simulink model "scale_model_model_control"  (R2024b)
settings: Solver=VariableStepAuto  StartTime=0.0  StopTime=100  MaxStep=0.02  RelTol=1e-3
values from neighbouring files (symbols this model uses):
  A_adrcl = [zeros(N, 1)  eye(N, N) ... (first row only)    [init_scale_blade_suspended_control.m]
  A_ESO_d = [1-l1_ESO_d, delta_t-l1_ESO_d*delta_t, 1/2 * delta_t^2 - 1/2 * l1_ESO_d*delta_t^2 ... (first row only)    [init_scale_blade_suspended_control.m]
  A_MESO_d = A_o_d - l_MESO_d*C_o_d*A_o_d    [init_scale_blade_suspended_control.m]
  b0 = 1.025    [init_scale_blade_suspended_control.m]
  b_adrcl = [zeros(N-1, 1) ... (first row only)    [init_scale_blade_suspended_control.m]
  b_ESO_d = [1/2*b0*delta_t^2 - l1_ESO_d*b0*delta_t^2 ... (first row only)    [init_scale_blade_suspended_control.m]
  B_MESO_d = B_o_d - l_MESO_d*C_o_d*B_o_d    [init_scale_blade_suspended_control.m]
  c_t = [1, zeros(1, N)]    [init_scale_blade_suspended_control.m]
  delta_t = 0.01    [init_scale_blade_suspended_control.m]
  DLADRC_max_effort = 30    [init_scale_blade_suspended_control.m]
  DLQRMADRC_max_effort = 30    [init_scale_blade_suspended_control.m]
  eta_s_init_n = [p_s_init_n;Theta_s_init_n]    [init_scale_blade_suspended_control.m]
  g = 9.81    [init_scale_blade_suspended_control.m]
  inv_M_s = inv(M_s)    [init_scale_blade_suspended_control.m]
  k = ones(N,1)    [init_scale_blade_suspended_control.m]
  k1_c_d = (1 - z_cl)^2/delta_t^2    [init_scale_blade_suspended_control.m]
  k_c_T_dlqr = dlqr(A_m_dlqr,b_m_dlqr,Q,R)    [init_scale_blade_suspended_control.m]
  k_d_T_lqr = (e_m*c_T_d_m_lqr) \ b_m_lqr    [init_scale_blade_suspended_control.m]
  k_s_lqr = -inv(c_T_m_lqr*inv(A_m_lqr-b_m_lqr*k_c_T_lqr)*b_m_lqr)    [init_scale_blade_suspended_control.m]
  k_T_d = [k1_c_d, k2_c_d]    [init_scale_blade_suspended_control.m]
  k_w1_s = gamma * EA/lw1_s_init    (= 19634.9540849)    [init_scale_blade_suspended_control.m]
  k_w2_s = k_w1_s    (= 19634.9540849)    [init_scale_blade_suspended_control.m]
  L = 0.8    [init_scale_blade_suspended_control.m]
  l = ones(N+1, 1)    [init_scale_blade_suspended_control.m]
  l_ESO_d = [l1_ESO_d, l2_ESO_d, l3_ESO_d]'    [init_scale_blade_suspended_control.m]
  l_MESO_d = acker(A_o_d',C_o_d',[z_MESO,z_MESO,z_MESO])'    [init_scale_blade_suspended_control.m]
  lw1_s_init = tot_liftWire-0.14    (= 0.56)    [init_scale_blade_suspended_control.m]
  lw2_s = norm(p_h_s_init- posSling_s_n(:,1))-elong_lw2_s    [init_scale_blade_suspended_control.m]
  m_h_s = 0.01    [init_scale_blade_suspended_control.m]
  meanWSP = 1    [init_scale_blade_suspended_control.m]
  N = 2    [init_scale_blade_suspended_control.m]
  nu_s_init_b = zeros(6,1)    [init_scale_blade_suspended_control.m]
  p_h_dot_s_init = [0;0;0]    [init_scale_blade_suspended_control.m]
  p_h_s_init = posCraneTip_s + [0;0;lw1_s_init + elong_mainlw_s]    [init_scale_blade_suspended_control.m]
  posCOG_s = [0;0;0]    [init_scale_blade_suspended_control.m]
  posCraneTip_s = [0;0;-1.2]    [init_scale_blade_suspended_control.m]
  posSling_s_b = [posCOG_s + [slings_p1_new(1); -0.05; slings_p1_new(2)],                posCOG_s + [slings_p1_new(1); 0.05; slings_p1_new(2)],               posCOG_s + [slings_p2_new(1); -0.05; slings_p2_new(2)],               posCOG_s + [slings_p2_new(1); 0.05; slings_p2_new(2)]]    [init_scale_blade_suspended_control.m]
  posThruster_s_b = [posCOG_s + [0.03; 0.21; -0.05],                posCOG_s + [0.03; -0.21; -0.05],               posCOG_s + [0; 0.1825; -0.05],               posCOG_s + [0; -0.1825; -0.05]]    [init_scale_blade_suspended_control.m]
  totalMass_s = 0.391    [init_scale_blade_suspended_control.m]
  W = 0.05    [init_scale_blade_suspended_control.m]
undefined symbols (not defined in the file or in its folder): A_o_dlqr, b_o_dlqr, c_o_T_dlqr, k_o_lqr, linsys_v2, sigbuilder_block
libraries: MarIn_blade x104, simulink_extras x28, slpidlib x5, simulink x4
(part 1 of 3)
settings Model: Creator=Basti  LastModifiedBy=Henrik
settings DebuggingCC: UnconnectedInputMsg=warning  UnconnectedOutputMsg=warning  UnconnectedLineMsg=warning
settings ModelReferenceCC: EnableRefExpFcnMdlSchedulingChecks=on
settings RTWCC: GPUComputeCapability=3.5  DLArmComputeVersion=19.05

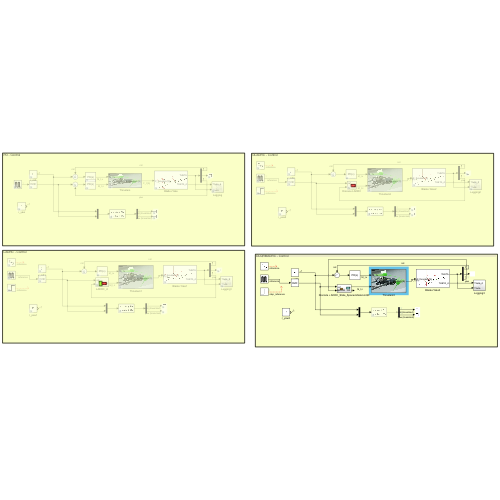
[thumbnail: Simulink's stored preview of the top-level diagram]
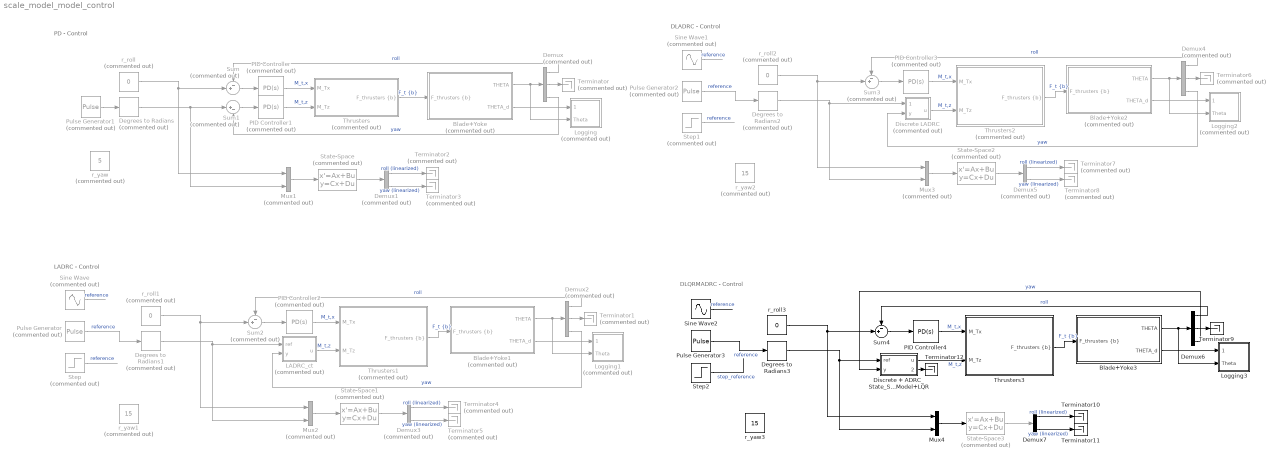
== system scale_model_model_control ==
  note: PD - Control
  note: LADRC - Control
  note: DLADRC - Control
  note: DLQRMADRC - Control
  Blade+Yoke : Subsystem  Commented=on
      mask Display: image('$imagefile'); % Use "Edit Image" on toolstrip to change.
  Blade+Yoke1 : Subsystem  Commented=on
      mask Display: image('$imagefile'); % Use "Edit Image" on toolstrip to change.
  Blade+Yoke2 : Subsystem  Commented=on
      mask Display: image('$imagefile'); % Use "Edit Image" on toolstrip to change.
  Blade+Yoke3 : Subsystem
      mask Display: image('$imagefile'); % Use "Edit Image" on toolstrip to change.
  Degrees to Radians : simulink_extras/Transformations/Degrees to Radians  Commented=on
  Degrees to Radians1 : simulink_extras/Transformations/Degrees to Radians  Commented=on
  Degrees to Radians2 : simulink_extras/Transformations/Degrees to Radians  Commented=on
  Degrees to Radians3 : simulink_extras/Transformations/Degrees to Radians
  Demux : Demux  Commented=on  Outputs=3
  Demux1 : Demux  Commented=on  Outputs=2
  Demux2 : Demux  Commented=on  Outputs=3
  Demux3 : Demux  Commented=on  Outputs=2
  Demux4 : Demux  Commented=on  Outputs=3
  Demux5 : Demux  Commented=on  Outputs=2
  Demux6 : Demux  Outputs=3
  Demux7 : Demux  Outputs=2
  Discrete + ADRC_State_Space+Model+LQR : Subsystem
  Discrete LADRC : Subsystem  Commented=on
  LADRC_ct : Subsystem  Commented=on
  Logging : Subsystem  Commented=on
  Logging1 : Subsystem  Commented=on
  Logging2 : Subsystem  Commented=on
  Logging3 : Subsystem
  Mux1 : Mux  Commented=on  Inputs=2
  Mux2 : Mux  Commented=on  Inputs=2
  Mux3 : Mux  Commented=on  Inputs=2
  Mux4 : Mux  Inputs=2
  PID Controller : slpidlib/PID Controller  Commented=on  Controller=PD  Form=Parallel  TimeDomain=Continuous-time  UseExternalTs=off  SampleTime=-1  IntegratorMethod=Forward Euler  FilterMethod=Forward Euler  ControllerParametersSource=internal  P=0.561459634219398  I=1  UseKiTs=off  D=0.260333020296235  UseExternalDerivativeSource=off  N=93.2588541333035  UseFilter=on  TunerSelectOption=Transfer Function Based (PID Tuner App)  InitialConditionSource=internal  InitialConditionForIntegrator=0  InitialConditionForFilter=0  DifferentiatorICPrevScaledInput=0  ExternalReset=none  TrackingMode=off  Kt=1  LimitOutput=off  SatLimitsSource=internal  UpperSaturationLimit=inf  LowerSaturationLimit=-inf  LinearizeAsGain=on  AntiWindupMode=none  Kb=1  LimitIntegrator=off  UpperIntegratorSaturationLimit=inf  LowerIntegratorSaturationLimit=-inf  POutMin=[]  POutMax=[]  IOutMin=[]  IOutMax=[]  DOutMin=[]  DOutMax=[]  NOutMin=[]  NOutMax=[]  SumOutMin=[]  SumOutMax=[]  SaturationOutMin=[]  SaturationOutMax=[]  PParamMin=[]  PParamMax=[]  IParamMin=[]  IParamMax=[]  DParamMin=[]  DParamMax=[]  NParamMin=[]  NParamMax=[]  KbParamMin=[]  KbParamMax=[]  KtParamMin=[]  KtParamMax=[]  KbOutMin=[]  KbOutMax=[]  KtOutMin=[]  KtOutMax=[]  IntegratorOutMin=[]  IntegratorOutMax=[]  FilterOutMin=[]  FilterOutMax=[]  SumI1OutMin=[]  SumI1OutMax=[]  SumI2OutMin=[]  SumI2OutMax=[]  SumI3OutMin=[]  SumI3OutMax=[]  SumI4OutMin=[]  SumI4OutMax=[]  SumDOutMin=[]  SumDOutMax=[]  DifferentiatorOutMin=[]  DifferentiatorOutMax=[]  FilterDiffOutCoefMin=[]  FilterDiffOutCoefMax=[]  ReciprocalOutMin=[]  ReciprocalOutMax=[]  SumDenOutMin=[]  SumDenOutMax=[]  SumNumOutMin=[]  SumNumOutMax=[]  DivideOutMin=[]  DivideOutMax=[]  UdiffTsProdOutMin=[]  UdiffTsProdOutMax=[]  NTsProdOutMin=[]  NTsProdOutMax=[]  UintegralTsProdOutMin=[]  UintegralTsProdOutMax=[]  UngainTsProdOutMin=[]  UngainTsProdOutMax=[]  ClampingZeroOutDataTypeStr=Inherit: Inherit via back propagation  ClampingZeroOutMin=[]  ClampingZeroOutMax=[]  FilterDenConstantOutDataTypeStr=Inherit: Inherit via back propagation  FilterDenConstantOutMin=[]  FilterDenConstantOutMax=[]  PCopyOutDataTypeStr=Inherit: Inherit via back propagation  PCopyOutMin=[]  PCopyOutMax=[]  NCopyOutDataTypeStr=Inherit: Inherit via back propagation  NCopyOutMin=[]  NCopyOutMax=[]  IntegratorContinuousStateAttributes=''  IntegratorStateMustResolveToSignalObject=off  IntegratorRTWStateStorageClass=Auto  FilterContinuousStateAttributes=''  FilterStateMustResolveToSignalObject=off  FilterRTWStateStorageClass=Auto  ParallelPVariant=InternalParameters  IdealPVariant=Disabled  IVariant=Disabled  DVariant=InternalParameters  IntegratorVariant=Disabled  SatVariant=Disabled  AWVariant=Disabled  PCopyVariant=Disabled  TRVariant=Disabled  FdbkBlocksVariant=Forward  IdealPFdbkVariant=Disabled  SatFdbkVariant=Disabled  DerivativeFilterVariant=ContFilter  NVariant=InternalParameters  NCopyVariant=Disabled  FilterICVariant=InternalICsFilter  IntegratorICVariant=Disabled  ExternalResetVariant=Disabled  TRSumVariant=Passthrough  SumFdbkVariant=Disabled  SumVariant=Sum_PD  TsampFilterVariant=InternalTs  TsampNgainVariant=Passthrough  TsampIntegralVariant=Disabled_SignalSpec  ExternalSaturationOutDataTypeStr=Inherit: Same as second input  DerivativeSourceVariant=ErrorSignal  PreIntVariant=InternalPreInt
  PID Controller1 : slpidlib/PID Controller  Commented=on  Controller=PD  Form=Parallel  TimeDomain=Continuous-time  UseExternalTs=off  SampleTime=-1  IntegratorMethod=Forward Euler  FilterMethod=Forward Euler  ControllerParametersSource=internal  P=12.7  I=1  UseKiTs=off  D=1.297*5  UseExternalDerivativeSource=off  N=6677.648  UseFilter=on  TunerSelectOption=Transfer Function Based (PID Tuner App)  InitialConditionSource=internal  InitialConditionForIntegrator=0  InitialConditionForFilter=0  DifferentiatorICPrevScaledInput=0  ExternalReset=none  TrackingMode=off  Kt=1  LimitOutput=off  SatLimitsSource=internal  UpperSaturationLimit=inf  LowerSaturationLimit=-inf  LinearizeAsGain=on  AntiWindupMode=none  Kb=1  LimitIntegrator=off  UpperIntegratorSaturationLimit=inf  LowerIntegratorSaturationLimit=-inf  POutMin=[]  POutMax=[]  IOutMin=[]  IOutMax=[]  DOutMin=[]  DOutMax=[]  NOutMin=[]  NOutMax=[]  SumOutMin=[]  SumOutMax=[]  SaturationOutMin=[]  SaturationOutMax=[]  PParamMin=[]  PParamMax=[]  IParamMin=[]  IParamMax=[]  DParamMin=[]  DParamMax=[]  NParamMin=[]  NParamMax=[]  KbParamMin=[]  KbParamMax=[]  KtParamMin=[]  KtParamMax=[]  KbOutMin=[]  KbOutMax=[]  KtOutMin=[]  KtOutMax=[]  IntegratorOutMin=[]  IntegratorOutMax=[]  FilterOutMin=[]  FilterOutMax=[]  SumI1OutMin=[]  SumI1OutMax=[]  SumI2OutMin=[]  SumI2OutMax=[]  SumI3OutMin=[]  SumI3OutMax=[]  SumI4OutMin=[]  SumI4OutMax=[]  SumDOutMin=[]  SumDOutMax=[]  DifferentiatorOutMin=[]  DifferentiatorOutMax=[]  FilterDiffOutCoefMin=[]  FilterDiffOutCoefMax=[]  ReciprocalOutMin=[]  ReciprocalOutMax=[]  SumDenOutMin=[]  SumDenOutMax=[]  SumNumOutMin=[]  SumNumOutMax=[]  DivideOutMin=[]  DivideOutMax=[]  UdiffTsProdOutMin=[]  UdiffTsProdOutMax=[]  NTsProdOutMin=[]  NTsProdOutMax=[]  UintegralTsProdOutMin=[]  UintegralTsProdOutMax=[]  UngainTsProdOutMin=[]  UngainTsProdOutMax=[]  ClampingZeroOutDataTypeStr=Inherit: Inherit via back propagation  ClampingZeroOutMin=[]  ClampingZeroOutMax=[]  FilterDenConstantOutDataTypeStr=Inherit: Inherit via back propagation  FilterDenConstantOutMin=[]  FilterDenConstantOutMax=[]  PCopyOutDataTypeStr=Inherit: Inherit via back propagation  PCopyOutMin=[]  PCopyOutMax=[]  NCopyOutDataTypeStr=Inherit: Inherit via back propagation  NCopyOutMin=[]  NCopyOutMax=[]  IntegratorContinuousStateAttributes=''  IntegratorStateMustResolveToSignalObject=off  IntegratorRTWStateStorageClass=Auto  FilterContinuousStateAttributes=''  FilterStateMustResolveToSignalObject=off  FilterRTWStateStorageClass=Auto  ParallelPVariant=InternalParameters  IdealPVariant=Disabled  IVariant=Disabled  DVariant=InternalParameters  IntegratorVariant=Disabled  SatVariant=Disabled  AWVariant=Disabled  PCopyVariant=Disabled  TRVariant=Disabled  FdbkBlocksVariant=Forward  IdealPFdbkVariant=Disabled  SatFdbkVariant=Disabled  DerivativeFilterVariant=ContFilter  NVariant=InternalParameters  NCopyVariant=Disabled  FilterICVariant=InternalICsFilter  IntegratorICVariant=Disabled  ExternalResetVariant=Disabled  TRSumVariant=Passthrough  SumFdbkVariant=Disabled  SumVariant=Sum_PD  TsampFilterVariant=InternalTs  TsampNgainVariant=Passthrough  TsampIntegralVariant=Disabled_SignalSpec  ExternalSaturationOutDataTypeStr=Inherit: Same as second input  DerivativeSourceVariant=ErrorSignal  PreIntVariant=InternalPreInt
  PID Controller2 : slpidlib/PID Controller  Commented=on  Controller=PD  Form=Parallel  TimeDomain=Continuous-time  UseExternalTs=off  SampleTime=-1  IntegratorMethod=Forward Euler  FilterMethod=Forward Euler  ControllerParametersSource=internal  P=0.561459634219398  I=1  UseKiTs=off  D=0.260333020296235  UseExternalDerivativeSource=off  N=93.2588541333035  UseFilter=on  TunerSelectOption=Transfer Function Based (PID Tuner App)  InitialConditionSource=internal  InitialConditionForIntegrator=0  InitialConditionForFilter=0  DifferentiatorICPrevScaledInput=0  ExternalReset=none  TrackingMode=off  Kt=1  LimitOutput=off  SatLimitsSource=internal  UpperSaturationLimit=inf  LowerSaturationLimit=-inf  LinearizeAsGain=on  AntiWindupMode=none  Kb=1  LimitIntegrator=off  UpperIntegratorSaturationLimit=inf  LowerIntegratorSaturationLimit=-inf  POutMin=[]  POutMax=[]  IOutMin=[]  IOutMax=[]  DOutMin=[]  DOutMax=[]  NOutMin=[]  NOutMax=[]  SumOutMin=[]  SumOutMax=[]  SaturationOutMin=[]  SaturationOutMax=[]  PParamMin=[]  PParamMax=[]  IParamMin=[]  IParamMax=[]  DParamMin=[]  DParamMax=[]  NParamMin=[]  NParamMax=[]  KbParamMin=[]  KbParamMax=[]  KtParamMin=[]  KtParamMax=[]  KbOutMin=[]  KbOutMax=[]  KtOutMin=[]  KtOutMax=[]  IntegratorOutMin=[]  IntegratorOutMax=[]  FilterOutMin=[]  FilterOutMax=[]  SumI1OutMin=[]  SumI1OutMax=[]  SumI2OutMin=[]  SumI2OutMax=[]  SumI3OutMin=[]  SumI3OutMax=[]  SumI4OutMin=[]  SumI4OutMax=[]  SumDOutMin=[]  SumDOutMax=[]  DifferentiatorOutMin=[]  DifferentiatorOutMax=[]  FilterDiffOutCoefMin=[]  FilterDiffOutCoefMax=[]  ReciprocalOutMin=[]  ReciprocalOutMax=[]  SumDenOutMin=[]  SumDenOutMax=[]  SumNumOutMin=[]  SumNumOutMax=[]  DivideOutMin=[]  DivideOutMax=[]  UdiffTsProdOutMin=[]  UdiffTsProdOutMax=[]  NTsProdOutMin=[]  NTsProdOutMax=[]  UintegralTsProdOutMin=[]  UintegralTsProdOutMax=[]  UngainTsProdOutMin=[]  UngainTsProdOutMax=[]  ClampingZeroOutDataTypeStr=Inherit: Inherit via back propagation  ClampingZeroOutMin=[]  ClampingZeroOutMax=[]  FilterDenConstantOutDataTypeStr=Inherit: Inherit via back propagation  FilterDenConstantOutMin=[]  FilterDenConstantOutMax=[]  PCopyOutDataTypeStr=Inherit: Inherit via back propagation  PCopyOutMin=[]  PCopyOutMax=[]  NCopyOutDataTypeStr=Inherit: Inherit via back propagation  NCopyOutMin=[]  NCopyOutMax=[]  IntegratorContinuousStateAttributes=''  IntegratorStateMustResolveToSignalObject=off  IntegratorRTWStateStorageClass=Auto  FilterContinuousStateAttributes=''  FilterStateMustResolveToSignalObject=off  FilterRTWStateStorageClass=Auto  ParallelPVariant=InternalParameters  IdealPVariant=Disabled  IVariant=Disabled  DVariant=InternalParameters  IntegratorVariant=Disabled  SatVariant=Disabled  AWVariant=Disabled  PCopyVariant=Disabled  TRVariant=Disabled  FdbkBlocksVariant=Forward  IdealPFdbkVariant=Disabled  SatFdbkVariant=Disabled  DerivativeFilterVariant=ContFilter  NVariant=InternalParameters  NCopyVariant=Disabled  FilterICVariant=InternalICsFilter  IntegratorICVariant=Disabled  ExternalResetVariant=Disabled  TRSumVariant=Passthrough  SumFdbkVariant=Disabled  SumVariant=Sum_PD  TsampFilterVariant=InternalTs  TsampNgainVariant=Passthrough  TsampIntegralVariant=Disabled_SignalSpec  ExternalSaturationOutDataTypeStr=Inherit: Same as second input  DerivativeSourceVariant=ErrorSignal  PreIntVariant=InternalPreInt
  PID Controller3 : slpidlib/PID Controller  Commented=on  Controller=PD  Form=Parallel  TimeDomain=Continuous-time  UseExternalTs=off  SampleTime=-1  IntegratorMethod=Forward Euler  FilterMethod=Forward Euler  ControllerParametersSource=internal  P=0.561459634219398  I=1  UseKiTs=off  D=0.260333020296235  UseExternalDerivativeSource=off  N=93.2588541333035  UseFilter=on  TunerSelectOption=Transfer Function Based (PID Tuner App)  InitialConditionSource=internal  InitialConditionForIntegrator=0  InitialConditionForFilter=0  DifferentiatorICPrevScaledInput=0  ExternalReset=none  TrackingMode=off  Kt=1  LimitOutput=off  SatLimitsSource=internal  UpperSaturationLimit=inf  LowerSaturationLimit=-inf  LinearizeAsGain=on  AntiWindupMode=none  Kb=1  LimitIntegrator=off  UpperIntegratorSaturationLimit=inf  LowerIntegratorSaturationLimit=-inf  POutMin=[]  POutMax=[]  IOutMin=[]  IOutMax=[]  DOutMin=[]  DOutMax=[]  NOutMin=[]  NOutMax=[]  SumOutMin=[]  SumOutMax=[]  SaturationOutMin=[]  SaturationOutMax=[]  PParamMin=[]  PParamMax=[]  IParamMin=[]  IParamMax=[]  DParamMin=[]  DParamMax=[]  NParamMin=[]  NParamMax=[]  KbParamMin=[]  KbParamMax=[]  KtParamMin=[]  KtParamMax=[]  KbOutMin=[]  KbOutMax=[]  KtOutMin=[]  KtOutMax=[]  IntegratorOutMin=[]  IntegratorOutMax=[]  FilterOutMin=[]  FilterOutMax=[]  SumI1OutMin=[]  SumI1OutMax=[]  SumI2OutMin=[]  SumI2OutMax=[]  SumI3OutMin=[]  SumI3OutMax=[]  SumI4OutMin=[]  SumI4OutMax=[]  SumDOutMin=[]  SumDOutMax=[]  DifferentiatorOutMin=[]  DifferentiatorOutMax=[]  FilterDiffOutCoefMin=[]  FilterDiffOutCoefMax=[]  ReciprocalOutMin=[]  ReciprocalOutMax=[]  SumDenOutMin=[]  SumDenOutMax=[]  SumNumOutMin=[]  SumNumOutMax=[]  DivideOutMin=[]  DivideOutMax=[]  UdiffTsProdOutMin=[]  UdiffTsProdOutMax=[]  NTsProdOutMin=[]  NTsProdOutMax=[]  UintegralTsProdOutMin=[]  UintegralTsProdOutMax=[]  UngainTsProdOutMin=[]  UngainTsProdOutMax=[]  ClampingZeroOutDataTypeStr=Inherit: Inherit via back propagation  ClampingZeroOutMin=[]  ClampingZeroOutMax=[]  FilterDenConstantOutDataTypeStr=Inherit: Inherit via back propagation  FilterDenConstantOutMin=[]  FilterDenConstantOutMax=[]  PCopyOutDataTypeStr=Inherit: Inherit via back propagation  PCopyOutMin=[]  PCopyOutMax=[]  NCopyOutDataTypeStr=Inherit: Inherit via back propagation  NCopyOutMin=[]  NCopyOutMax=[]  IntegratorContinuousStateAttributes=''  IntegratorStateMustResolveToSignalObject=off  IntegratorRTWStateStorageClass=Auto  FilterContinuousStateAttributes=''  FilterStateMustResolveToSignalObject=off  FilterRTWStateStorageClass=Auto  ParallelPVariant=InternalParameters  IdealPVariant=Disabled  IVariant=Disabled  DVariant=InternalParameters  IntegratorVariant=Disabled  SatVariant=Disabled  AWVariant=Disabled  PCopyVariant=Disabled  TRVariant=Disabled  FdbkBlocksVariant=Forward  IdealPFdbkVariant=Disabled  SatFdbkVariant=Disabled  DerivativeFilterVariant=ContFilter  NVariant=InternalParameters  NCopyVariant=Disabled  FilterICVariant=InternalICsFilter  IntegratorICVariant=Disabled  ExternalResetVariant=Disabled  TRSumVariant=Passthrough  SumFdbkVariant=Disabled  SumVariant=Sum_PD  TsampFilterVariant=InternalTs  TsampNgainVariant=Passthrough  TsampIntegralVariant=Disabled_SignalSpec  ExternalSaturationOutDataTypeStr=Inherit: Same as second input  DerivativeSourceVariant=ErrorSignal  PreIntVariant=InternalPreInt
  PID Controller4 : slpidlib/PID Controller  Controller=PD  Form=Parallel  TimeDomain=Continuous-time  UseExternalTs=off  SampleTime=-1  IntegratorMethod=Forward Euler  FilterMethod=Forward Euler  ControllerParametersSource=internal  P=0.561459634219398  I=1  UseKiTs=off  D=0.260333020296235  UseExternalDerivativeSource=off  N=93.2588541333035  UseFilter=on  TunerSelectOption=Transfer Function Based (PID Tuner App)  InitialConditionSource=internal  InitialConditionForIntegrator=0  InitialConditionForFilter=0  DifferentiatorICPrevScaledInput=0  ExternalReset=none  TrackingMode=off  Kt=1  LimitOutput=off  SatLimitsSource=internal  UpperSaturationLimit=inf  LowerSaturationLimit=-inf  LinearizeAsGain=on  AntiWindupMode=none  Kb=1  LimitIntegrator=off  UpperIntegratorSaturationLimit=inf  LowerIntegratorSaturationLimit=-inf  POutMin=[]  POutMax=[]  IOutMin=[]  IOutMax=[]  DOutMin=[]  DOutMax=[]  NOutMin=[]  NOutMax=[]  SumOutMin=[]  SumOutMax=[]  SaturationOutMin=[]  SaturationOutMax=[]  PParamMin=[]  PParamMax=[]  IParamMin=[]  IParamMax=[]  DParamMin=[]  DParamMax=[]  NParamMin=[]  NParamMax=[]  KbParamMin=[]  KbParamMax=[]  KtParamMin=[]  KtParamMax=[]  KbOutMin=[]  KbOutMax=[]  KtOutMin=[]  KtOutMax=[]  IntegratorOutMin=[]  IntegratorOutMax=[]  FilterOutMin=[]  FilterOutMax=[]  SumI1OutMin=[]  SumI1OutMax=[]  SumI2OutMin=[]  SumI2OutMax=[]  SumI3OutMin=[]  SumI3OutMax=[]  SumI4OutMin=[]  SumI4OutMax=[]  SumDOutMin=[]  SumDOutMax=[]  DifferentiatorOutMin=[]  DifferentiatorOutMax=[]  FilterDiffOutCoefMin=[]  FilterDiffOutCoefMax=[]  ReciprocalOutMin=[]  ReciprocalOutMax=[]  SumDenOutMin=[]  SumDenOutMax=[]  SumNumOutMin=[]  SumNumOutMax=[]  DivideOutMin=[]  DivideOutMax=[]  UdiffTsProdOutMin=[]  UdiffTsProdOutMax=[]  NTsProdOutMin=[]  NTsProdOutMax=[]  UintegralTsProdOutMin=[]  UintegralTsProdOutMax=[]  UngainTsProdOutMin=[]  UngainTsProdOutMax=[]  ClampingZeroOutDataTypeStr=Inherit: Inherit via back propagation  ClampingZeroOutMin=[]  ClampingZeroOutMax=[]  FilterDenConstantOutDataTypeStr=Inherit: Inherit via back propagation  FilterDenConstantOutMin=[]  FilterDenConstantOutMax=[]  PCopyOutDataTypeStr=Inherit: Inherit via back propagation  PCopyOutMin=[]  PCopyOutMax=[]  NCopyOutDataTypeStr=Inherit: Inherit via back propagation  NCopyOutMin=[]  NCopyOutMax=[]  IntegratorContinuousStateAttributes=''  IntegratorStateMustResolveToSignalObject=off  IntegratorRTWStateStorageClass=Auto  FilterContinuousStateAttributes=''  FilterStateMustResolveToSignalObject=off  FilterRTWStateStorageClass=Auto  ParallelPVariant=InternalParameters  IdealPVariant=Disabled  IVariant=Disabled  DVariant=InternalParameters  IntegratorVariant=Disabled  SatVariant=Disabled  AWVariant=Disabled  PCopyVariant=Disabled  TRVariant=Disabled  FdbkBlocksVariant=Forward  IdealPFdbkVariant=Disabled  SatFdbkVariant=Disabled  DerivativeFilterVariant=ContFilter  NVariant=InternalParameters  NCopyVariant=Disabled  FilterICVariant=InternalICsFilter  IntegratorICVariant=Disabled  ExternalResetVariant=Disabled  TRSumVariant=Passthrough  SumFdbkVariant=Disabled  SumVariant=Sum_PD  TsampFilterVariant=InternalTs  TsampNgainVariant=Passthrough  TsampIntegralVariant=Disabled_SignalSpec  ExternalSaturationOutDataTypeStr=Inherit: Same as second input  DerivativeSourceVariant=ErrorSignal  PreIntVariant=InternalPreInt
  Pulse Generator : DiscretePulseGenerator  Commented=on  PulseType=Time based  Amplitude=50  Period=20  PulseWidth=50  PhaseDelay=5
  Pulse Generator1 : DiscretePulseGenerator  Commented=on  PulseType=Time based  Amplitude=50  Period=20  PulseWidth=50  PhaseDelay=5
  Pulse Generator2 : DiscretePulseGenerator  Commented=on  PulseType=Time based  Amplitude=50  Period=20  PulseWidth=50  PhaseDelay=5
  Pulse Generator3 : DiscretePulseGenerator  PulseType=Time based  Amplitude=90  Period=60  PulseWidth=50  PhaseDelay=5
  Sine Wave : Sin  Commented=on  Amplitude=15  Frequency=0.05*2*pi  SampleTime=0
  Sine Wave1 : Sin  Commented=on  Amplitude=15  Frequency=0.05*2*pi  SampleTime=0
  Sine Wave2 : Sin  Amplitude=15  Frequency=0.05*2*pi  SampleTime=0
  State-Space{,1..3} (4 alike) : StateSpace  Commented=on  A=linsys_v2.A  B=linsys_v2.B  C=linsys_v2.C  D=linsys_v2.D  InitialCondition=0
  Step : Step  Commented=on  Time=5  After=15  SampleTime=0
  Step1 : Step  Commented=on  Time=5  After=15  SampleTime=0
  Step2 : Step  Time=5  After=15  SampleTime=0
  Sum : Sum  Commented=on  Inputs=-+|
  Sum1 : Sum  Commented=on  Inputs=|+-
  Sum2 : Sum  Commented=on  Inputs=-+|
  Sum3 : Sum  Commented=on  Inputs=-+|
  Sum4 : Sum  Inputs=-+|
  Terminator{,1..8} (9 alike) : Terminator  Commented=on
  Terminator{9..12} (4 alike) : Terminator
  Thrusters : Subsystem  Commented=on
      mask Display: image('$imagefile'); % Use "Edit Image" on toolstrip to change.
  Thrusters1 : Subsystem  Commented=on
      mask Display: image('$imagefile'); % Use "Edit Image" on toolstrip to change.
  Thrusters2 : Subsystem  Commented=on
      mask Display: image('$imagefile'); % Use "Edit Image" on toolstrip to change.
  Thrusters3 : Subsystem
      mask Display: image('$imagefile'); % Use "Edit Image" on toolstrip to change.
  r_roll : Constant  Commented=on  Value=0
  r_roll1 : Constant  Commented=on  Value=0
  r_roll2 : Constant  Commented=on  Value=0
  r_roll3 : Constant  Value=0
  r_yaw : Constant  Commented=on  Value=5
  r_yaw1 : Constant  Commented=on  Value=15
  r_yaw2 : Constant  Commented=on  Value=15
  r_yaw3 : Constant  Value=15
  wires:
  Blade+Yoke/1(THETA) -> Demux/1, Logging/2(Theta)
  Demux/3 -> Sum1/2  "yaw"
  Demux/1 -> Sum/1  "roll"
  Degrees to Radians/1 -> Mux1/2, Sum1/1
  r_roll/1 -> Mux1/1, Sum/2
  Thrusters/1("F_thrusters {b}") -> Blade+Yoke/1("F_thrusters {b}")  "F_t {b}"
  Sum/1 -> PID Controller/1
  Sum1/1 -> PID Controller1/1
  PID Controller/1 -> Thrusters/1(M_Tx)  "M_t,x"
  PID Controller1/1 -> Thrusters/2(M_Tz)  "M_t,z"
  Blade+Yoke/2(THETA_d) -> Logging/1(Theta_d)
  Demux/2 -> Terminator/1
  Mux1/1 -> State-Space/1
  State-Space/1 -> Demux1/1
  Demux1/1 -> Terminator2/1  "roll (linearized)"
  Demux1/2 -> Terminator3/1  "yaw (linearized)"
  Degrees to Radians1/1 -> Mux2/2, LADRC_ct/1(ref)
  Pulse Generator/1 -> Degrees to Radians1/1  "reference"
  LADRC_ct/1(u) -> Thrusters1/2(M_Tz)  "M_t,z"
  Blade+Yoke1/2(THETA_d) -> Logging1/1(Theta_d)
  Mux2/1 -> State-Space1/1
  Demux3/2 -> Terminator5/1  "yaw (linearized)"
  Demux3/1 -> Terminator4/1  "roll (linearized)"
  Blade+Yoke1/1(THETA) -> Demux2/1, Logging1/2(Theta)
  Sum2/1 -> PID Controller2/1
  Demux2/1 -> Sum2/1  "roll"
  State-Space1/1 -> Demux3/1
  r_roll1/1 -> Mux2/1, Sum2/2
  Demux2/2 -> Terminator1/1
  Thrusters1/1("F_thrusters {b}") -> Blade+Yoke1/1("F_thrusters {b}")  "F_t {b}"
  PID Controller2/1 -> Thrusters1/1(M_Tx)  "M_t,x"
  Demux2/3 -> LADRC_ct/2(y)  "yaw"
  Sine Wave/1 -> ?  "reference"
  Step/1 -> ?  "reference"
  Pulse Generator1/1 -> Degrees to Radians/1
  r_roll2/1 -> Mux3/1, Sum3/2
  Demux5/2 -> Terminator8/1  "yaw (linearized)"
  Sum3/1 -> PID Controller3/1
  Pulse Generator2/1 -> Degrees to Radians2/1  "reference"
  Degrees to Radians2/1 -> Discrete LADRC/1(ref), Mux3/2
  Blade+Yoke2/2(THETA_d) -> Logging2/1(Theta_d)
  Demux4/3 -> Discrete LADRC/2(y)  "yaw"
  PID Controller3/1 -> Thrusters2/1(M_Tx)  "M_t,x"
  State-Space2/1 -> Demux5/1
  Demux5/1 -> Terminator7/1  "roll (linearized)"
  Demux4/2 -> Terminator6/1
  Thrusters2/1("F_thrusters {b}") -> Blade+Yoke2/1("F_thrusters {b}")  "F_t {b}"
  Sine Wave1/1 -> ?  "reference"
  Step1/1 -> ?  "reference"
  Demux4/1 -> Sum3/1  "roll"
  Blade+Yoke2/1(THETA) -> Demux4/1, Logging2/2(Theta)
  Mux3/1 -> State-Space2/1
  Discrete LADRC/1(u) -> Thrusters2/2(M_Tz)  "M_t,z"
  Demux6/3 -> Discrete + ADRC_State_Space+Model+LQR/2(y)  "yaw"
  Sum4/1 -> PID Controller4/1
  Demux6/2 -> Terminator9/1
  PID Controller4/1 -> Thrusters3/1(M_Tx)  "M_t,x"
  Thrusters3/1("F_thrusters {b}") -> Blade+Yoke3/1("F_thrusters {b}")  "F_t {b}"
  r_roll3/1 -> Mux4/1, Sum4/2
  Blade+Yoke3/1(THETA) -> Demux6/1, Logging3/2(Theta)
  Mux4/1 -> State-Space3/1
  Blade+Yoke3/2(THETA_d) -> Logging3/1(Theta_d)
  Degrees to Radians3/1 -> Discrete + ADRC_State_Space+Model+LQR/1(ref), Mux4/2
  Demux7/1 -> Terminator10/1  "roll (linearized)"
  State-Space3/1 -> Demux7/1
  Demux6/1 -> Sum4/1  "roll"
  Step2/1 -> ?  "step_reference"
  Sine Wave2/1 -> ?  "reference"
  Discrete + ADRC_State_Space+Model+LQR/1(u) -> Thrusters3/2(M_Tz)  "M_t,z"
  Pulse Generator3/1 -> Degrees to Radians3/1  "reference"
  Demux7/2 -> Terminator11/1  "yaw (linearized)"
  Discrete + ADRC_State_Space+Model+LQR/2(ESO+M - out) -> Terminator12/1

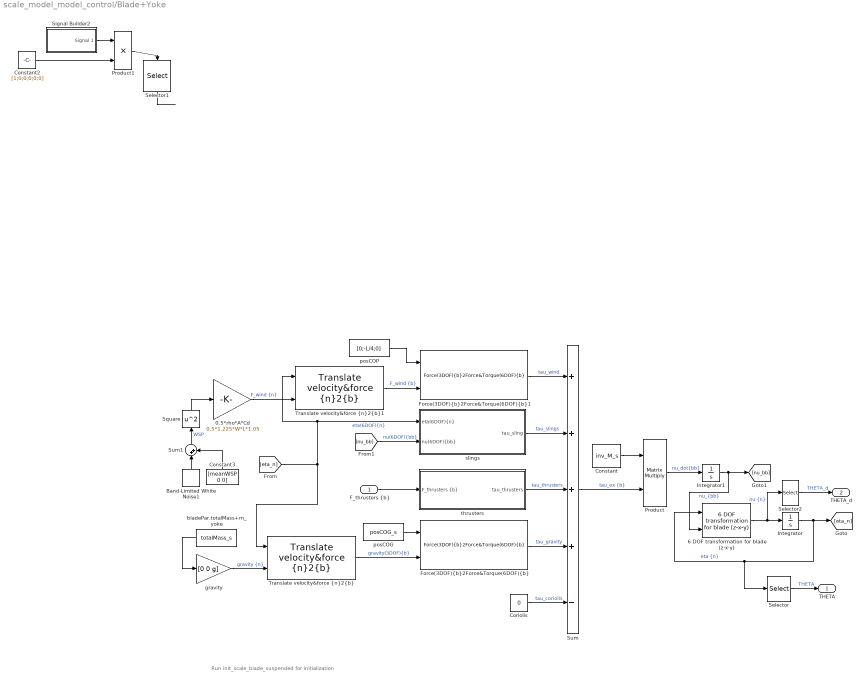
== system scale_model_model_control/Blade+Yoke ==
  note: Run init_scale_blade_suspended for initialization
  "F_thrusters {b}" : Inport
  0.5*rho*A*Cd : Gain  Gain=0.5*1.225*W*L*1.05
  6 DOF transformation for blade (z-x-y) : MarIn_blade/Basic functions/6 DOF transformation for blade (z-x-y)
      settings: SourceProductName=MarIn (Blade)
  Band-Limited White Noise1 : simulink/Sources/Band-Limited White Noise  Cov=[0.001 0.001 0.001]  Ts=0.1  seed=[23321 232341 23441]
  Constant : Constant  Value=inv_M_s
  Constant2 : Constant  Value=[1;0;0;0;0;0]
  Constant3 : Constant  Value=[meanWSP 0 0]
  Coriolis : Constant  Value=0
  "Force(3DOF){b}2Force&Torque(6DOF){b}" : MarIn_blade/Basic functions/Force(3DOF){b}2Force&Torque(6DOF){b}  posCOG_bb=posCOG_s
      settings: SourceProductName=MarIn (Blade)
  "Force(3DOF){b}2Force&Torque(6DOF){b}1" : MarIn_blade/Basic functions/Force(3DOF){b}2Force&Torque(6DOF){b}  posCOG_bb=posCOG_s
      settings: SourceProductName=MarIn (Blade)
  Integrator : Integrator  InitialCondition=eta_s_init_n  ContinuousStateAttributes='eta_n'
  "Integrator1 " : Integrator  InitialCondition=nu_s_init_b  ContinuousStateAttributes='nu_b'
  Product : Product  Inputs=**  Multiplication=Matrix(*)
  Product1 : Product
  Selector : Selector  InputPortWidth=6  IndexOptions=Index vector (dialog)  Indices=[4 5 6]  OutputSizes=1
  Selector1 : Selector  InputPortWidth=6  IndexOptions=Index vector (dialog)  Indices=[1 2 3]  OutputSizes=1
  Selector2 : Selector  InputPortWidth=6  IndexOptions=Index vector (dialog)  Indices=[4 5 6]  OutputSizes=1
  Signal Builder2 : Subsystem  Tag=STV Subsys  LoadFcn=sigbuilder_block('load');  StartFcn=sigbuilder_block('start');  StopFcn=sigbuilder_block('stop');  ClipboardFcn=sigbuilder_block('clipboard');  mask(Sigbuilder block){tuvar=[0:10]}
      mask help: Simulink:masks:SigbuilderBlock_MD
      mask init:
      | if ~strcmp(get_param(bdroot(gcbh),'SimulationStatus'),'stopped') tuvar = sigbuilder_block('maskInit'); end
      settings: CopyFcn=sigbuilder_block('copy');  DeleteFcn=sigbuilder_block('delete');  ModelCloseFcn=sigbuilder_block('modelClose');  PreSaveFcn=sigbuilder_block('preSave');  PauseFcn=sigbuilder_block('pause');  ContinueFcn=sigbuilder_block('continue');  NameChangeFcn=sigbuilder_block('namechange');  OpenFcn=sigbuilder_block('open',[437.6 199.2 550.4 400 ]);  CloseFcn=sigbuilder_block('close');
      mask Display: plot(0, 0, 100, 100,[2, 2, 32, 32, 2], [68, 8, 8, 68, 68],[32, 2], [38, 38], [32, 19, 2],[53, 60, 44], [32, 17, 17, 2],[16, 16, 31, 31]);txt = getActiveGroup(gcbh);text(2, 100, txt,'verticalAlignment', 'top');
  Square : Math  Operator=square
  Sum : Sum  Inputs=++++-
  Sum1 : Sum  Inputs=|++
  "Translate velocity&force {n}2{b}" : MarIn_blade/Basic functions/Translate velocity&force {n}2{b}
      settings: SourceProductName=MarIn (Blade)
  "Translate velocity&force {n}2{b}1" : MarIn_blade/Basic functions/Translate velocity&force {n}2{b}
      settings: SourceProductName=MarIn (Blade)
  bladePar.totalMass+m_yoke : Constant  Value=totalMass_s
  gravity : Gain  Gain=[0 0 g]
  posCOG : Constant  Value=posCOG_s
  posCOP : Constant  Value=[0;-L/4;0]
  slings : Subsystem
  thrusters : Subsystem
  THETA : Outport
  THETA_d : Outport  Port=2
  wires:
  Coriolis/1 -> Sum/5  "tau_coriolis"
  6 DOF transformation for blade (z-x-y)/1 -> Integrator/1, Selector2/1  "nu {n}"
  "Translate velocity&force {n}2{b}"/1 -> "Force(3DOF){b}2Force&Torque(6DOF){b}"/2  "gravity(3DOF){b}"
  "Integrator1 "/1 -> [nu_bb], 6 DOF transformation for blade (z-x-y)/2  "nu_{bb}"
  "F_thrusters {b}"/1 -> thrusters/1("F_thrusters {b}")
  Sum/1 -> Product/2  "tau_ex {b}"
  Product/1 -> "Integrator1 "/1  "nu_dot{bb}"
  Integrator/1 -> [eta_n], Selector/1, 6 DOF transformation for blade (z-x-y)/1  "eta {n}"
  "Force(3DOF){b}2Force&Torque(6DOF){b}"/1 -> Sum/4  "tau_gravity"
  [eta_n] -> slings/1("eta(6DOF){n}"), "Translate velocity&force {n}2{b}1"/1, "Translate velocity&force {n}2{b}"/1  "eta(6DOF){n}"
  slings/1(tau_sling) -> Sum/2  "tau_slings"
  Constant/1 -> Product/1
  gravity/1 -> "Translate velocity&force {n}2{b}"/2  "gravity {n}"
  thrusters/1(tau_thrusters) -> Sum/3  "tau_thrusters"
  bladePar.totalMass+m_yoke/1 -> gravity/1
  [nu_bb] -> slings/2("nu(6DOF){bb}")  "nu(6DOF){bb}"
  posCOG/1 -> "Force(3DOF){b}2Force&Torque(6DOF){b}"/1
  Selector/1 -> THETA/1  "THETA"
  Constant2/1 -> Product1/2
  Signal Builder2/1(Signal 1) -> Product1/1
  posCOP/1 -> "Force(3DOF){b}2Force&Torque(6DOF){b}1"/1
  "Force(3DOF){b}2Force&Torque(6DOF){b}1"/1 -> Sum/1  "tau_wind"
  0.5*rho*A*Cd/1 -> "Translate velocity&force {n}2{b}1"/2  "F_wind {n}"
  Square/1 -> 0.5*rho*A*Cd/1
  Sum1/1 -> Square/1  "WSP"
  Constant3/1 -> Sum1/2
  "Translate velocity&force {n}2{b}1"/1 -> "Force(3DOF){b}2Force&Torque(6DOF){b}1"/2  "F_wind {b}"
  Product1/1 -> Selector1/1
  Selector1/1 -> ?
  Selector2/1 -> THETA_d/1  "THETA_d"
  Band-Limited White Noise1/1 -> Sum1/1

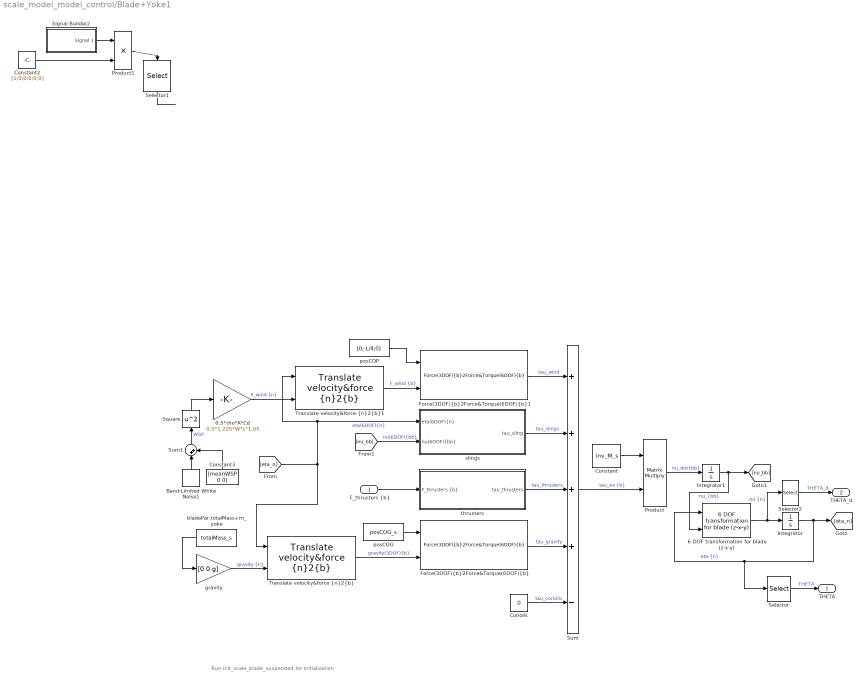
== system scale_model_model_control/Blade+Yoke1 ==
  note: Run init_scale_blade_suspended for initialization
  "F_thrusters {b}" : Inport
  0.5*rho*A*Cd : Gain  Gain=0.5*1.225*W*L*1.05
  6 DOF transformation for blade (z-x-y) : MarIn_blade/Basic functions/6 DOF transformation for blade (z-x-y)
      settings: SourceProductName=MarIn (Blade)
  Band-Limited White Noise1 : simulink/Sources/Band-Limited White Noise  Cov=[0.001 0.001 0.001]  Ts=0.1  seed=[23321 232341 23441]
  Constant : Constant  Value=inv_M_s
  Constant2 : Constant  Value=[1;0;0;0;0;0]
  Constant3 : Constant  Value=[meanWSP 0 0]
  Coriolis : Constant  Value=0
  "Force(3DOF){b}2Force&Torque(6DOF){b}" : MarIn_blade/Basic functions/Force(3DOF){b}2Force&Torque(6DOF){b}  posCOG_bb=posCOG_s
      settings: SourceProductName=MarIn (Blade)
  "Force(3DOF){b}2Force&Torque(6DOF){b}1" : MarIn_blade/Basic functions/Force(3DOF){b}2Force&Torque(6DOF){b}  posCOG_bb=posCOG_s
      settings: SourceProductName=MarIn (Blade)
  Integrator : Integrator  InitialCondition=eta_s_init_n  ContinuousStateAttributes='eta_n'
  "Integrator1 " : Integrator  InitialCondition=nu_s_init_b  ContinuousStateAttributes='nu_b'
  Product : Product  Inputs=**  Multiplication=Matrix(*)
  Product1 : Product
  Selector : Selector  InputPortWidth=6  IndexOptions=Index vector (dialog)  Indices=[4 5 6]  OutputSizes=1
  Selector1 : Selector  InputPortWidth=6  IndexOptions=Index vector (dialog)  Indices=[1 2 3]  OutputSizes=1
  Selector2 : Selector  InputPortWidth=6  IndexOptions=Index vector (dialog)  Indices=[4 5 6]  OutputSizes=1
  Signal Builder2 : Subsystem  Tag=STV Subsys  LoadFcn=sigbuilder_block('load');  StartFcn=sigbuilder_block('start');  StopFcn=sigbuilder_block('stop');  ClipboardFcn=sigbuilder_block('clipboard');  mask(Sigbuilder block){tuvar=[0:10]}
      mask help: Simulink:masks:SigbuilderBlock_MD
      mask init:
      | if ~strcmp(get_param(bdroot(gcbh),'SimulationStatus'),'stopped') tuvar = sigbuilder_block('maskInit'); end
      settings: CopyFcn=sigbuilder_block('copy');  DeleteFcn=sigbuilder_block('delete');  ModelCloseFcn=sigbuilder_block('modelClose');  PreSaveFcn=sigbuilder_block('preSave');  PauseFcn=sigbuilder_block('pause');  ContinueFcn=sigbuilder_block('continue');  NameChangeFcn=sigbuilder_block('namechange');  OpenFcn=sigbuilder_block('open',[437.6 199.2 550.4 400 ]);  CloseFcn=sigbuilder_block('close');
      mask Display: plot(0, 0, 100, 100,[2, 2, 32, 32, 2], [68, 8, 8, 68, 68],[32, 2], [38, 38], [32, 19, 2],[53, 60, 44], [32, 17, 17, 2],[16, 16, 31, 31]);txt = getActiveGroup(gcbh);text(2, 100, txt,'verticalAlignment', 'top');
  Square : Math  Operator=square
  Sum : Sum  Inputs=++++-
  Sum1 : Sum  Inputs=|++
  "Translate velocity&force {n}2{b}" : MarIn_blade/Basic functions/Translate velocity&force {n}2{b}
      settings: SourceProductName=MarIn (Blade)
  "Translate velocity&force {n}2{b}1" : MarIn_blade/Basic functions/Translate velocity&force {n}2{b}
      settings: SourceProductName=MarIn (Blade)
  bladePar.totalMass+m_yoke : Constant  Value=totalMass_s
  gravity : Gain  Gain=[0 0 g]
  posCOG : Constant  Value=posCOG_s
  posCOP : Constant  Value=[0;-L/4;0]
  slings : Subsystem
  thrusters : Subsystem
  THETA : Outport
  THETA_d : Outport  Port=2
  wires:
  Coriolis/1 -> Sum/5  "tau_coriolis"
  6 DOF transformation for blade (z-x-y)/1 -> Integrator/1, Selector2/1  "nu {n}"
  "Translate velocity&force {n}2{b}"/1 -> "Force(3DOF){b}2Force&Torque(6DOF){b}"/2  "gravity(3DOF){b}"
  "Integrator1 "/1 -> [nu_bb], 6 DOF transformation for blade (z-x-y)/2  "nu_{bb}"
  "F_thrusters {b}"/1 -> thrusters/1("F_thrusters {b}")
  Sum/1 -> Product/2  "tau_ex {b}"
  Product/1 -> "Integrator1 "/1  "nu_dot{bb}"
  Integrator/1 -> [eta_n], Selector/1, 6 DOF transformation for blade (z-x-y)/1  "eta {n}"
  "Force(3DOF){b}2Force&Torque(6DOF){b}"/1 -> Sum/4  "tau_gravity"
  [eta_n] -> slings/1("eta(6DOF){n}"), "Translate velocity&force {n}2{b}1"/1, "Translate velocity&force {n}2{b}"/1  "eta(6DOF){n}"
  slings/1(tau_sling) -> Sum/2  "tau_slings"
  Constant/1 -> Product/1
  gravity/1 -> "Translate velocity&force {n}2{b}"/2  "gravity {n}"
  thrusters/1(tau_thrusters) -> Sum/3  "tau_thrusters"
  bladePar.totalMass+m_yoke/1 -> gravity/1
  [nu_bb] -> slings/2("nu(6DOF){bb}")  "nu(6DOF){bb}"
  posCOG/1 -> "Force(3DOF){b}2Force&Torque(6DOF){b}"/1
  Selector/1 -> THETA/1  "THETA"
  Constant2/1 -> Product1/2
  Signal Builder2/1(Signal 1) -> Product1/1
  posCOP/1 -> "Force(3DOF){b}2Force&Torque(6DOF){b}1"/1
  "Force(3DOF){b}2Force&Torque(6DOF){b}1"/1 -> Sum/1  "tau_wind"
  0.5*rho*A*Cd/1 -> "Translate velocity&force {n}2{b}1"/2  "F_wind {n}"
  Square/1 -> 0.5*rho*A*Cd/1
  Sum1/1 -> Square/1  "WSP"
  Constant3/1 -> Sum1/2
  "Translate velocity&force {n}2{b}1"/1 -> "Force(3DOF){b}2Force&Torque(6DOF){b}1"/2  "F_wind {b}"
  Product1/1 -> Selector1/1
  Selector1/1 -> ?
  Selector2/1 -> THETA_d/1  "THETA_d"
  Band-Limited White Noise1/1 -> Sum1/1

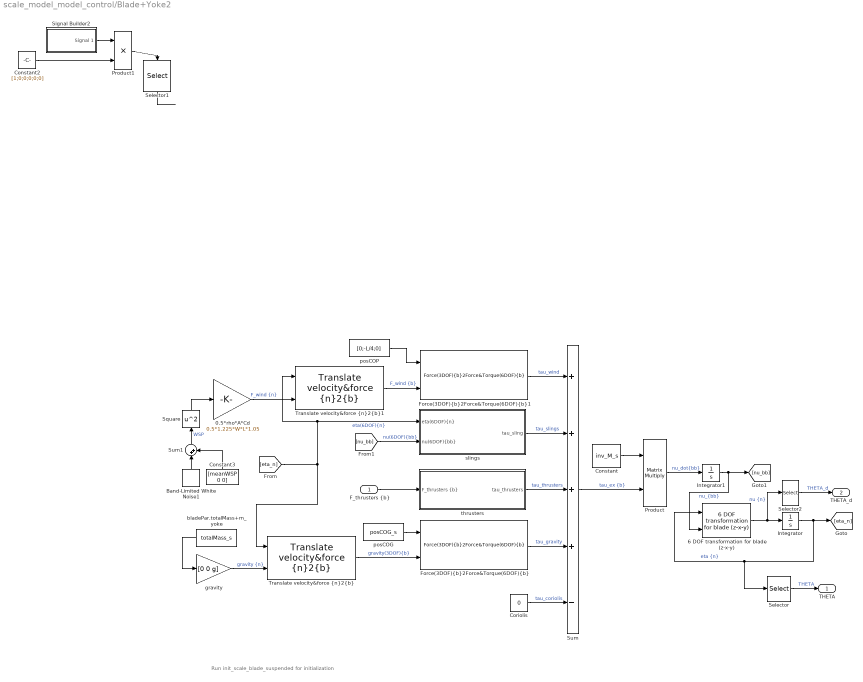
== system scale_model_model_control/Blade+Yoke2 ==
  note: Run init_scale_blade_suspended for initialization
  "F_thrusters {b}" : Inport
  0.5*rho*A*Cd : Gain  Gain=0.5*1.225*W*L*1.05
  6 DOF transformation for blade (z-x-y) : MarIn_blade/Basic functions/6 DOF transformation for blade (z-x-y)
      settings: SourceProductName=MarIn (Blade)
  Band-Limited White Noise1 : simulink/Sources/Band-Limited White Noise  Cov=[0.001 0.001 0.001]  Ts=0.1  seed=[23321 232341 23441]
  Constant : Constant  Value=inv_M_s
  Constant2 : Constant  Value=[1;0;0;0;0;0]
  Constant3 : Constant  Value=[meanWSP 0 0]
  Coriolis : Constant  Value=0
  "Force(3DOF){b}2Force&Torque(6DOF){b}" : MarIn_blade/Basic functions/Force(3DOF){b}2Force&Torque(6DOF){b}  posCOG_bb=posCOG_s
      settings: SourceProductName=MarIn (Blade)
  "Force(3DOF){b}2Force&Torque(6DOF){b}1" : MarIn_blade/Basic functions/Force(3DOF){b}2Force&Torque(6DOF){b}  posCOG_bb=posCOG_s
      settings: SourceProductName=MarIn (Blade)
  Integrator : Integrator  InitialCondition=eta_s_init_n  ContinuousStateAttributes='eta_n'
  "Integrator1 " : Integrator  InitialCondition=nu_s_init_b  ContinuousStateAttributes='nu_b'
  Product : Product  Inputs=**  Multiplication=Matrix(*)
  Product1 : Product
  Selector : Selector  InputPortWidth=6  IndexOptions=Index vector (dialog)  Indices=[4 5 6]  OutputSizes=1
  Selector1 : Selector  InputPortWidth=6  IndexOptions=Index vector (dialog)  Indices=[1 2 3]  OutputSizes=1
  Selector2 : Selector  InputPortWidth=6  IndexOptions=Index vector (dialog)  Indices=[4 5 6]  OutputSizes=1
  Signal Builder2 : Subsystem  Tag=STV Subsys  LoadFcn=sigbuilder_block('load');  StartFcn=sigbuilder_block('start');  StopFcn=sigbuilder_block('stop');  ClipboardFcn=sigbuilder_block('clipboard');  mask(Sigbuilder block){tuvar=[0:10]}
      mask help: Simulink:masks:SigbuilderBlock_MD
      mask init:
      | if ~strcmp(get_param(bdroot(gcbh),'SimulationStatus'),'stopped') tuvar = sigbuilder_block('maskInit'); end
      settings: CopyFcn=sigbuilder_block('copy');  DeleteFcn=sigbuilder_block('delete');  ModelCloseFcn=sigbuilder_block('modelClose');  PreSaveFcn=sigbuilder_block('preSave');  PauseFcn=sigbuilder_block('pause');  ContinueFcn=sigbuilder_block('continue');  NameChangeFcn=sigbuilder_block('namechange');  OpenFcn=sigbuilder_block('open',[437.6 199.2 550.4 400 ]);  CloseFcn=sigbuilder_block('close');
      mask Display: plot(0, 0, 100, 100,[2, 2, 32, 32, 2], [68, 8, 8, 68, 68],[32, 2], [38, 38], [32, 19, 2],[53, 60, 44], [32, 17, 17, 2],[16, 16, 31, 31]);txt = getActiveGroup(gcbh);text(2, 100, txt,'verticalAlignment', 'top');
  Square : Math  Operator=square
  Sum : Sum  Inputs=++++-
  Sum1 : Sum  Inputs=|++
  "Translate velocity&force {n}2{b}" : MarIn_blade/Basic functions/Translate velocity&force {n}2{b}
      settings: SourceProductName=MarIn (Blade)
  "Translate velocity&force {n}2{b}1" : MarIn_blade/Basic functions/Translate velocity&force {n}2{b}
      settings: SourceProductName=MarIn (Blade)
  bladePar.totalMass+m_yoke : Constant  Value=totalMass_s
  gravity : Gain  Gain=[0 0 g]
  posCOG : Constant  Value=posCOG_s
  posCOP : Constant  Value=[0;-L/4;0]
  slings : Subsystem
  thrusters : Subsystem
  THETA : Outport
  THETA_d : Outport  Port=2
  wires:
  Coriolis/1 -> Sum/5  "tau_coriolis"
  6 DOF transformation for blade (z-x-y)/1 -> Integrator/1, Selector2/1  "nu {n}"
  "Translate velocity&force {n}2{b}"/1 -> "Force(3DOF){b}2Force&Torque(6DOF){b}"/2  "gravity(3DOF){b}"
  "Integrator1 "/1 -> [nu_bb], 6 DOF transformation for blade (z-x-y)/2  "nu_{bb}"
  "F_thrusters {b}"/1 -> thrusters/1("F_thrusters {b}")
  Sum/1 -> Product/2  "tau_ex {b}"
  Product/1 -> "Integrator1 "/1  "nu_dot{bb}"
  Integrator/1 -> [eta_n], Selector/1, 6 DOF transformation for blade (z-x-y)/1  "eta {n}"
  "Force(3DOF){b}2Force&Torque(6DOF){b}"/1 -> Sum/4  "tau_gravity"
  [eta_n] -> slings/1("eta(6DOF){n}"), "Translate velocity&force {n}2{b}1"/1, "Translate velocity&force {n}2{b}"/1  "eta(6DOF){n}"
  slings/1(tau_sling) -> Sum/2  "tau_slings"
  Constant/1 -> Product/1
  gravity/1 -> "Translate velocity&force {n}2{b}"/2  "gravity {n}"
  thrusters/1(tau_thrusters) -> Sum/3  "tau_thrusters"
  bladePar.totalMass+m_yoke/1 -> gravity/1
  [nu_bb] -> slings/2("nu(6DOF){bb}")  "nu(6DOF){bb}"
  posCOG/1 -> "Force(3DOF){b}2Force&Torque(6DOF){b}"/1
  Selector/1 -> THETA/1  "THETA"
  Constant2/1 -> Product1/2
  Signal Builder2/1(Signal 1) -> Product1/1
  posCOP/1 -> "Force(3DOF){b}2Force&Torque(6DOF){b}1"/1
  "Force(3DOF){b}2Force&Torque(6DOF){b}1"/1 -> Sum/1  "tau_wind"
  0.5*rho*A*Cd/1 -> "Translate velocity&force {n}2{b}1"/2  "F_wind {n}"
  Square/1 -> 0.5*rho*A*Cd/1
  Sum1/1 -> Square/1  "WSP"
  Constant3/1 -> Sum1/2
  "Translate velocity&force {n}2{b}1"/1 -> "Force(3DOF){b}2Force&Torque(6DOF){b}1"/2  "F_wind {b}"
  Product1/1 -> Selector1/1
  Selector1/1 -> ?
  Selector2/1 -> THETA_d/1  "THETA_d"
  Band-Limited White Noise1/1 -> Sum1/1

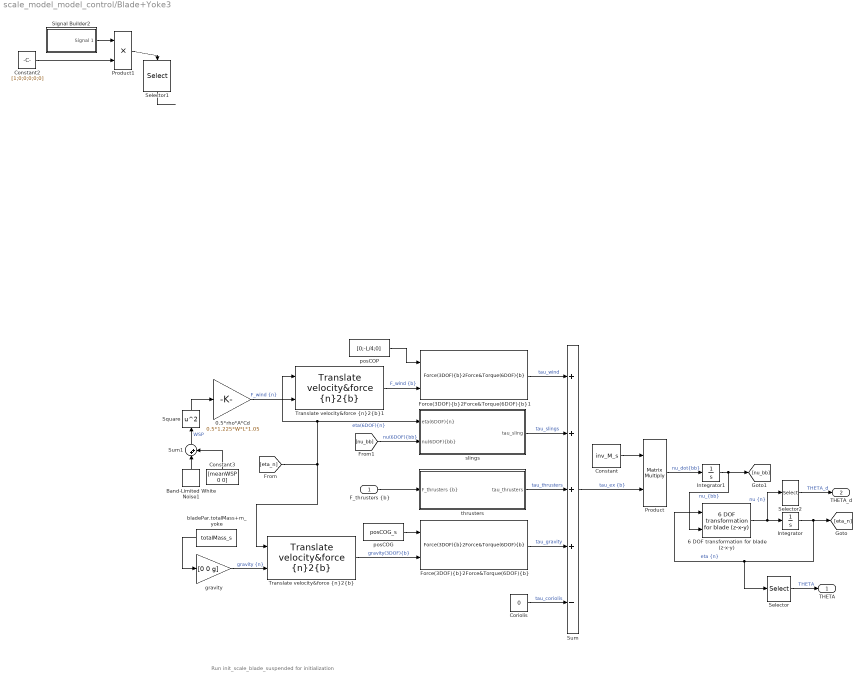
== system scale_model_model_control/Blade+Yoke3 ==
  note: Run init_scale_blade_suspended for initialization
  "F_thrusters {b}" : Inport
  0.5*rho*A*Cd : Gain  Gain=0.5*1.225*W*L*1.05
  6 DOF transformation for blade (z-x-y) : MarIn_blade/Basic functions/6 DOF transformation for blade (z-x-y)
      settings: SourceProductName=MarIn (Blade)
  Band-Limited White Noise1 : simulink/Sources/Band-Limited White Noise  Cov=[0.001 0.001 0.001]  Ts=0.1  seed=[23321 232341 23441]
  Constant : Constant  Value=inv_M_s
  Constant2 : Constant  Value=[1;0;0;0;0;0]
  Constant3 : Constant  Value=[meanWSP 0 0]
  Coriolis : Constant  Value=0
  "Force(3DOF){b}2Force&Torque(6DOF){b}" : MarIn_blade/Basic functions/Force(3DOF){b}2Force&Torque(6DOF){b}  posCOG_bb=posCOG_s
      settings: SourceProductName=MarIn (Blade)
  "Force(3DOF){b}2Force&Torque(6DOF){b}1" : MarIn_blade/Basic functions/Force(3DOF){b}2Force&Torque(6DOF){b}  posCOG_bb=posCOG_s
      settings: SourceProductName=MarIn (Blade)
  Integrator : Integrator  InitialCondition=eta_s_init_n  ContinuousStateAttributes='eta_n'
  "Integrator1 " : Integrator  InitialCondition=nu_s_init_b  ContinuousStateAttributes='nu_b'
  Product : Product  Inputs=**  Multiplication=Matrix(*)
  Product1 : Product
  Selector : Selector  InputPortWidth=6  IndexOptions=Index vector (dialog)  Indices=[4 5 6]  OutputSizes=1
  Selector1 : Selector  InputPortWidth=6  IndexOptions=Index vector (dialog)  Indices=[1 2 3]  OutputSizes=1
  Selector2 : Selector  InputPortWidth=6  IndexOptions=Index vector (dialog)  Indices=[4 5 6]  OutputSizes=1
  Signal Builder2 : Subsystem  Tag=STV Subsys  LoadFcn=sigbuilder_block('load');  StartFcn=sigbuilder_block('start');  StopFcn=sigbuilder_block('stop');  ClipboardFcn=sigbuilder_block('clipboard');  mask(Sigbuilder block){tuvar=[0:10]}
      mask help: Simulink:masks:SigbuilderBlock_MD
      mask init:
      | if ~strcmp(get_param(bdroot(gcbh),'SimulationStatus'),'stopped') tuvar = sigbuilder_block('maskInit'); end
      settings: CopyFcn=sigbuilder_block('copy');  DeleteFcn=sigbuilder_block('delete');  ModelCloseFcn=sigbuilder_block('modelClose');  PreSaveFcn=sigbuilder_block('preSave');  PauseFcn=sigbuilder_block('pause');  ContinueFcn=sigbuilder_block('continue');  NameChangeFcn=sigbuilder_block('namechange');  OpenFcn=sigbuilder_block('open',[437.6 199.2 550.4 400 ]);  CloseFcn=sigbuilder_block('close');
      mask Display: plot(0, 0, 100, 100,[2, 2, 32, 32, 2], [68, 8, 8, 68, 68],[32, 2], [38, 38], [32, 19, 2],[53, 60, 44], [32, 17, 17, 2],[16, 16, 31, 31]);txt = getActiveGroup(gcbh);text(2, 100, txt,'verticalAlignment', 'top');
  Square : Math  Operator=square
  Sum : Sum  Inputs=++++-
  Sum1 : Sum  Inputs=|++
  "Translate velocity&force {n}2{b}" : MarIn_blade/Basic functions/Translate velocity&force {n}2{b}
      settings: SourceProductName=MarIn (Blade)
  "Translate velocity&force {n}2{b}1" : MarIn_blade/Basic functions/Translate velocity&force {n}2{b}
      settings: SourceProductName=MarIn (Blade)
  bladePar.totalMass+m_yoke : Constant  Value=totalMass_s
  gravity : Gain  Gain=[0 0 g]
  posCOG : Constant  Value=posCOG_s
  posCOP : Constant  Value=[0;-L/4;0]
  slings : Subsystem
  thrusters : Subsystem
  THETA : Outport
  THETA_d : Outport  Port=2
  wires:
  Coriolis/1 -> Sum/5  "tau_coriolis"
  6 DOF transformation for blade (z-x-y)/1 -> Integrator/1, Selector2/1  "nu {n}"
  "Translate velocity&force {n}2{b}"/1 -> "Force(3DOF){b}2Force&Torque(6DOF){b}"/2  "gravity(3DOF){b}"
  "Integrator1 "/1 -> [nu_bb], 6 DOF transformation for blade (z-x-y)/2  "nu_{bb}"
  "F_thrusters {b}"/1 -> thrusters/1("F_thrusters {b}")
  Sum/1 -> Product/2  "tau_ex {b}"
  Product/1 -> "Integrator1 "/1  "nu_dot{bb}"
  Integrator/1 -> [eta_n], Selector/1, 6 DOF transformation for blade (z-x-y)/1  "eta {n}"
  "Force(3DOF){b}2Force&Torque(6DOF){b}"/1 -> Sum/4  "tau_gravity"
  [eta_n] -> slings/1("eta(6DOF){n}"), "Translate velocity&force {n}2{b}1"/1, "Translate velocity&force {n}2{b}"/1  "eta(6DOF){n}"
  slings/1(tau_sling) -> Sum/2  "tau_slings"
  Constant/1 -> Product/1
  gravity/1 -> "Translate velocity&force {n}2{b}"/2  "gravity {n}"
  thrusters/1(tau_thrusters) -> Sum/3  "tau_thrusters"
  bladePar.totalMass+m_yoke/1 -> gravity/1
  [nu_bb] -> slings/2("nu(6DOF){bb}")  "nu(6DOF){bb}"
  posCOG/1 -> "Force(3DOF){b}2Force&Torque(6DOF){b}"/1
  Selector/1 -> THETA/1  "THETA"
  Constant2/1 -> Product1/2
  Signal Builder2/1(Signal 1) -> Product1/1
  posCOP/1 -> "Force(3DOF){b}2Force&Torque(6DOF){b}1"/1
  "Force(3DOF){b}2Force&Torque(6DOF){b}1"/1 -> Sum/1  "tau_wind"
  0.5*rho*A*Cd/1 -> "Translate velocity&force {n}2{b}1"/2  "F_wind {n}"
  Square/1 -> 0.5*rho*A*Cd/1
  Sum1/1 -> Square/1  "WSP"
  Constant3/1 -> Sum1/2
  "Translate velocity&force {n}2{b}1"/1 -> "Force(3DOF){b}2Force&Torque(6DOF){b}1"/2  "F_wind {b}"
  Product1/1 -> Selector1/1
  Selector1/1 -> ?
  Selector2/1 -> THETA_d/1  "THETA_d"
  Band-Limited White Noise1/1 -> Sum1/1

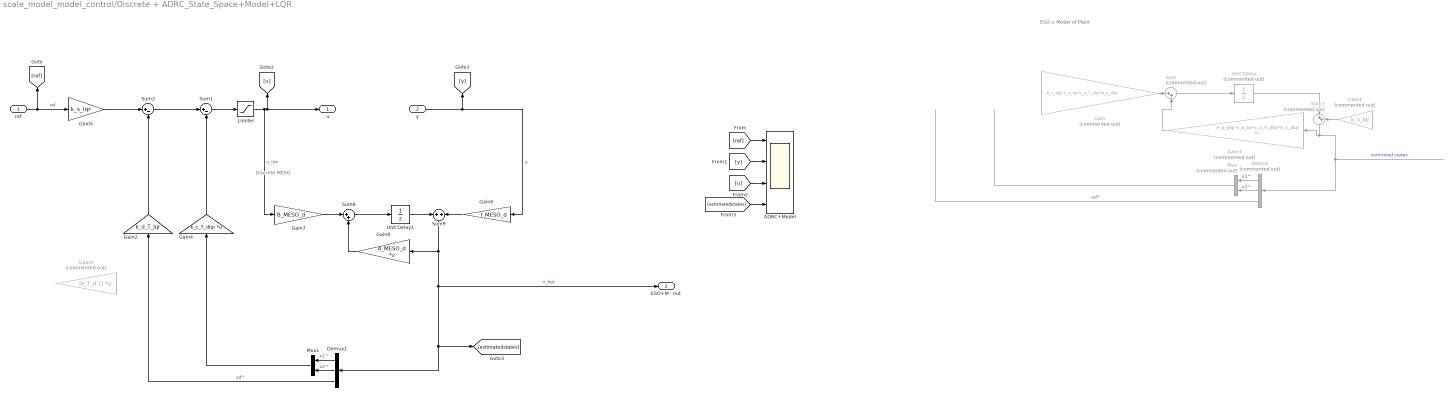
== system scale_model_model_control/Discrete + ADRC_State_Space+Model+LQR ==
  note: Discrete MESO
  note: ESO + Model of Plant
  ref : Inport
  y : Inport  Port=2
  ADRC+Model : Scope  NumInputPorts=4
  Demux : Demux  Commented=on  Outputs=N+1
  Demux1 : Demux  Outputs=N+1
  Gain : Gain  Commented=on  Gain=b_o_dlqr-k_o_lqr*c_o_T_dlqr*b_o_dlqr
  Gain1 : Gain  Commented=on  Gain=k_o_lqr
  Gain2 : Gain  Gain=k_d_T_lqr
  Gain3 : Gain  Commented=on  Gain=A_o_dlqr-k_o_lqr*c_o_T_dlqr*A_o_dlqr  Multiplication=Matrix(K*u)
  Gain4 : Gain  Gain=k_c_T_dlqr  Multiplication=Matrix(K*u)
  Gain5 : Gain  Gain=k_s_lqr
  Gain6 : Gain  Gain=l_MESO_d
  Gain7 : Gain  Gain=B_MESO_d
  Gain8 : Gain  Gain=A_MESO_d  Multiplication=Matrix(K*u)
  Gain9 : Gain  Commented=on  Gain=[k_T_d 1]  Multiplication=Matrix(K*u)
  Limiter : Saturate  UpperLimit=DLQRMADRC_max_effort  LowerLimit=-DLQRMADRC_max_effort
  Mux : Mux  Commented=on  Inputs=2
  Mux1 : Mux  Inputs=2
  Sum : Sum  Commented=on  Inputs=|++
  Sum1 : Sum  Inputs=|+-
  Sum2 : Sum  Inputs=|+-
  Sum3 : Sum  Commented=on  Inputs=|++
  Sum8 : Sum  Inputs=|++
  Sum9 : Sum  Inputs=+|+
  Unit Delay : UnitDelay  Commented=on  SampleTime=delta_t  HasFrameUpgradeWarning=on
  Unit Delay1 : UnitDelay  SampleTime=delta_t  HasFrameUpgradeWarning=on
  u : Outport
  ESO+M - out : Outport  Port=2
  wires:
  ref/1 -> Gain5/1, [ref]  "ref"
  y/1 -> Gain6/1, [y]  "y"
  [ref] -> ADRC+Model/1
  [y] -> ADRC+Model/2
  [u] -> ADRC+Model/3
  [estimatedstates] -> ADRC+Model/4
  Sum1/1 -> Limiter/1
  Gain4/1 -> Sum1/2
  Gain2/1 -> Sum2/2
  Sum2/1 -> Sum1/1
  Gain5/1 -> Sum2/1
  Sum8/1 -> Unit Delay1/1
  Gain8/1 -> Sum8/2
  Unit Delay1/1 -> Sum9/1
  Gain7/1 -> Sum8/1
  Limiter/1 -> u/1, [u], Gain7/1  "u_lim"
  Sum9/1 -> Demux1/1, [estimatedstates], ESO+M - out/1, Gain8/1  "x_hat"
  Gain6/1 -> Sum9/2
  Demux/3 -> ?  "xd^"
  Sum/1 -> Unit Delay/1
  Demux/2 -> Mux/2  "x2^"
  ? -> Gain/1  "u"
  Demux/1 -> Mux/1  "x1^"
  Sum3/1 -> Gain3/1, Demux/1  "estimated states"
  ? -> Gain1/1  "y"
  Mux/1 -> ?
  Unit Delay/1 -> Sum3/1
  Gain3/1 -> Sum/2
  Gain/1 -> Sum/1
  Gain1/1 -> Sum3/2
  Demux1/1 -> Mux1/1  "x1^"
  Mux1/1 -> Gain4/1
  Demux1/2 -> Mux1/2  "x2^"
  Demux1/3 -> Gain2/1  "xd^"
